simulink model "Lab_04_Task02"  (R2015a)
settings: Solver=ode45  StartTime=0.0  StopTime=10.0  RelTol=1e-3
libraries: cstblocks x4
settings Model: Creator=Amir  LastModifiedBy=Amir

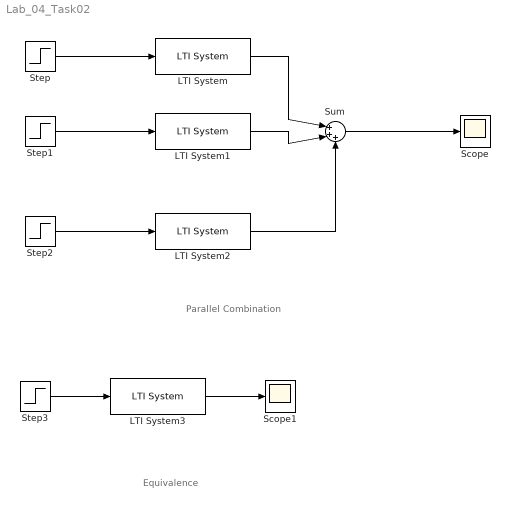
== system Lab_04_Task02 ==
  note: Equivalence
  note: Parallel Combination
  LTI System : cstblocks/LTI System  sys=tf(1,[1 1])  IC=[]
  LTI System1 : cstblocks/LTI System  sys=tf(1,[1 3])  IC=[]
  LTI System2 : cstblocks/LTI System  sys=tf([1 3],[1 5])  IC=[]
  LTI System3 : cstblocks/LTI System  sys=tf([1 9 29 29],[1 9 23 15])  IC=[]
  Scope : Scope
  Scope1 : Scope
  Step{,1..3} (4 alike) : Step  SampleTime=0
  Sum : Sum  Inputs=|+++
  wires:
  Step2/1 -> LTI System2/1
  Step1/1 -> LTI System1/1
  Step/1 -> LTI System/1
  Sum/1 -> Scope/1
  LTI System/1 -> Sum/1
  LTI System1/1 -> Sum/2
  LTI System2/1 -> Sum/3
  Step3/1 -> LTI System3/1
  LTI System3/1 -> Scope1/1
